simulink model "INP_ERR_test"  (R2024b)
settings: Solver=VariableStepAuto  StartTime=0.0  StopTime=10.0  RelTol=1e-3
libraries: simulink x1, INP_ERR x1
settings Model: Creator=blatak  LastModifiedBy=blatak

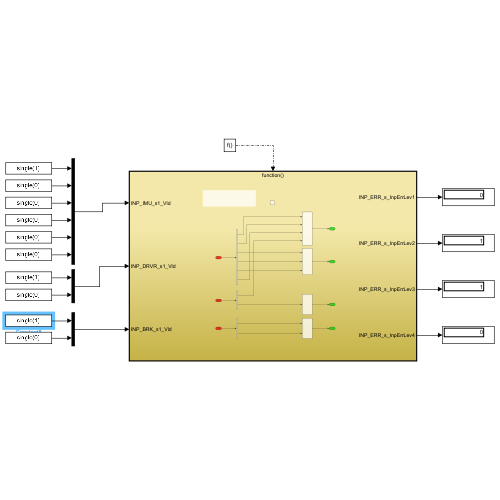
[thumbnail: Simulink's stored preview of the top-level diagram]
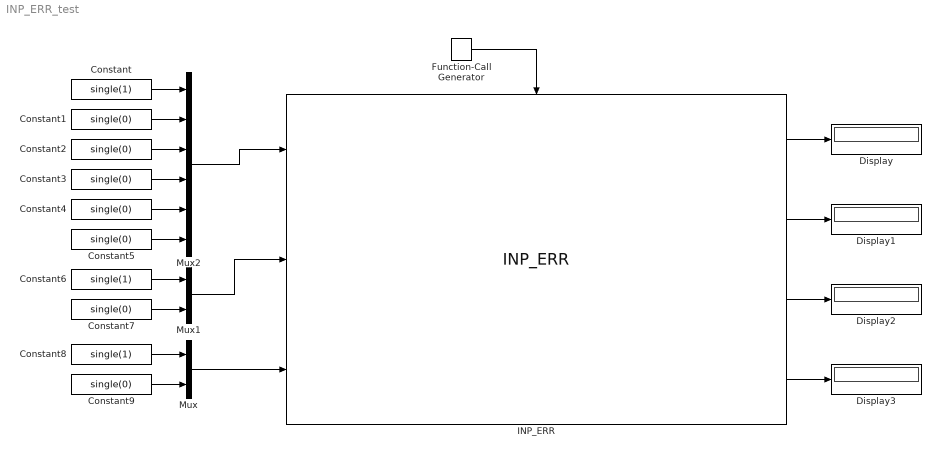
== system INP_ERR_test ==
  Constant : Constant  Value=single(1)
  Constant{1..5,7,9} (7 alike) : Constant  Value=single(0)
  Constant6 : Constant  Value=single(1)
  Constant8 : Constant  Value=single(1)
  Display{,1..3} (4 alike) : Display
  Function-Call Generator : simulink/Ports & Subsystems/Function-Call Generator  sample_time=0.005  numberOfIterations=1  DisallowWideOutput=off
  INP_ERR : INP_ERR/INP_ERR  SystemSampleTime=-1  VariantActivationTime=update diagram  AllowFlexibleInterface=on  Latency=0  AutoFrameSizeCalculation=off
  Mux : Mux  Inputs=2
  Mux1 : Mux  Inputs=2
  Mux2 : Mux  Inputs=6
  wires:
  Function-Call Generator/1 -> INP_ERR/Trigger
  INP_ERR/1 -> Display/1
  INP_ERR/2 -> Display1/1
  INP_ERR/3 -> Display2/1
  INP_ERR/4 -> Display3/1
  Constant8/1 -> Mux/1
  Constant9/1 -> Mux/2
  Constant6/1 -> Mux1/1
  Constant7/1 -> Mux1/2
  Mux1/1 -> INP_ERR/2
  Mux/1 -> INP_ERR/3
  Constant/1 -> Mux2/1
  Constant1/1 -> Mux2/2
  Constant2/1 -> Mux2/3
  Constant3/1 -> Mux2/4
  Constant4/1 -> Mux2/5
  Constant5/1 -> Mux2/6
  Mux2/1 -> INP_ERR/1
